simulink model "sgMdl_IO291_HS_DigitalLoopback"  (R2024b)
settings: Solver=FixedStepAuto  StartTime=0.0  StopTime=inf  RelTol=1e-3  EnableMultiTasking=on
undefined symbols (not defined in the file): HS, IO291
libraries: speedgoatlib_IO291 x5
Description:
  | IO291 HighSide - Digital LVTTL and FET Loopback
settings Model: ModifiedByFormat=Speedgoat  SimulationMode=external  ExtModeTrigDuration=100000  Creator=Speedgoat  LastModifiedBy=Speedgoat
settings SolverCC: ConcurrentTasks=on  AlgebraicLoopSolver=TrustRegion  PositivePriorityOrder=on  AutoInsertRateTranBlk=on
settings DataIOCC: LimitDataPoints=on  SaveFormat=StructureWithTime  ReturnWorkspaceOutputs=off
settings OptimizationCC: BlockReduction=off  OptimizeBlockIOStorage=off  BufferReuse=off  ReuseModelBlockBuffer=off  GlobalBufferReuse=off  ExpressionFolding=off  LocalBlockOutputs=off  OptimizeDataStoreBuffers=off  BusAssignmentInplaceUpdate=off
settings DebuggingCC: TasksWithSamePriorityMsg=none  UnconnectedInputMsg=warning  UnconnectedOutputMsg=warning  UnconnectedLineMsg=warning  AllowSymbolicDim=off  SFUnexpectedBacktrackingDiag=warning  SFNoUnconditionalDefaultTransitionDiag=warning  ArithmeticOperatorsInVariantConditions=warning
settings HardwareCC: ProdBitPerLong=64  ProdLongLongMode=on  ProdHWDeviceType=Intel->x86-64 (Linux 64)
settings ModelReferenceCC: EnableRefExpFcnMdlSchedulingChecks=on  PropagateSignalLabelsOutOfModel=off
settings SFSimCC: SimUseLocalCustomCode=off  CustomCodeUndefinedFunction=UseInterfaceOnly
settings RTWCC: Description=Speedgoat Real-Time Target Machine  SystemTargetFile=speedgoat.tlc  TemplateMakefile=slrealtime_default_tmf  RTWUseLocalCustomCode=off  Toolchain=Simulink Real-Time Toolchain  BuildConfiguration=Faster Runs  TargetLang=C++  GPUComputeCapability=3.5  DLArmComputeVersion=19.05
settings CodeAppCC: StateflowObjectComments=on
settings SimulinkRealTimeTargetCC: SubcomponentCodeInterfacePackaging=Reusable function  InstructionSetFMA=off  LogToMDFFile=off  SLRTFileLogMaxRuns=10  UseGCCFastMath=on
settings ConfigComp: CovMetricSettings=dw  CovSaveCumulativeToWorkspaceVar=on  CovSaveSingleToWorkspaceVar=on  CovExternalEMLEnable=off  CovBoundaryAbsTol=1.0e-5

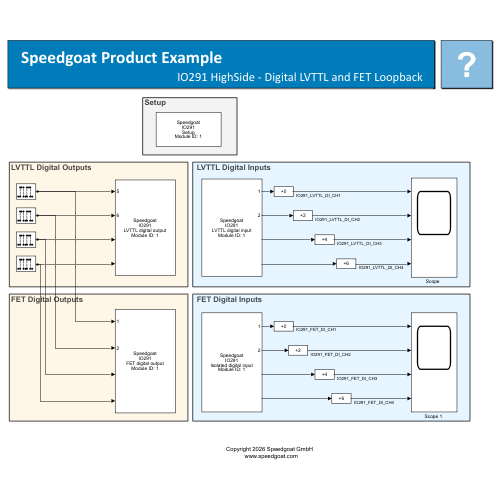
[thumbnail: Simulink's stored preview of the top-level diagram]
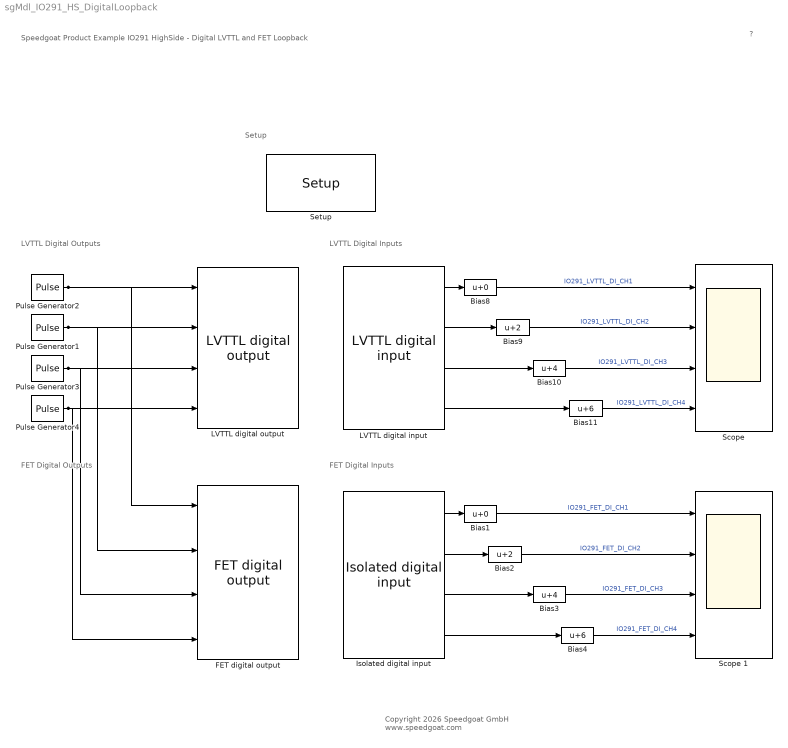
== system sgMdl_IO291_HS_DigitalLoopback ==
  note: LVTTL Digital Outputs
  note: LVTTL Digital Inputs
  note: Setup
  note: FET Digital Outputs
  note: FET Digital Inputs
  note: Speedgoat Product Example
      | IO291 HighSide - Digital LVTTL and FET Loopback
  note: ?
  note: Copyright 2026 Speedgoat GmbH
      |  www.speedgoat.com
  Bias1 : Bias  SaturateOnIntegerOverflow=off
  Bias10 : Bias  Bias=4  SaturateOnIntegerOverflow=off
  Bias11 : Bias  Bias=6  SaturateOnIntegerOverflow=off
  Bias2 : Bias  Bias=2  SaturateOnIntegerOverflow=off
  Bias3 : Bias  Bias=4  SaturateOnIntegerOverflow=off
  Bias4 : Bias  Bias=6  SaturateOnIntegerOverflow=off
  Bias8 : Bias  SaturateOnIntegerOverflow=off
  Bias9 : Bias  Bias=2  SaturateOnIntegerOverflow=off
  "FET digital output " : speedgoatlib_IO291/FET digital output   parModuleId=1  parSampleTime=0.01  parPortConf=1 port for each active output channel  parPciSlot=-1  parFetDoChannels=[1 2 3 4]  parFetDoInitValues=[0 0 0 0]  parFetDoReset=[1 1 1 1]  parModuleType=IO291-HS  parInternalModuleId=1
      settings: SourceProductName=Simulink Real-Time: Speedgoat I/O Blockset
  "Isolated digital input " : speedgoatlib_IO291/Isolated digital input   parModuleId=1  parSampleTime=0.01  parPortConf=1 port for each active input channel  parDataType=Double  parPciSlot=-1  parIsolDiChannels=[1 2 3 4]  parModuleType=IO291-HS  parInternalModuleId=1
      settings: SourceProductName=Simulink Real-Time: Speedgoat I/O Blockset
  "LVTTL digital input " : speedgoatlib_IO291/LVTTL digital input   parModuleId=1  parSampleTime=0.01  parPortConf=1 port for each active input channel  parDataType=Double  parPciSlot=-1  parTtlDiChannels=[1 2 3 4]  parModuleType=IO291-HS  parInternalModuleId=1
      settings: SourceProductName=Simulink Real-Time: Speedgoat I/O Blockset
  "LVTTL digital output " : speedgoatlib_IO291/LVTTL digital output   parModuleId=1  parSampleTime=0.01  parPortConf=1 port for each active output channel  parPciSlot=-1  parTtlDoChannels=[5 6 7 8]  parTtlDoInitValues=[0 0 0 0]  parTtlDoReset=[1 1 1 1]  parModuleType=IO291-HS  parInternalModuleId=1
      settings: SourceProductName=Simulink Real-Time: Speedgoat I/O Blockset
  Pulse Generator1 : DiscretePulseGenerator  Period=10  PulseWidth=4  SampleTime=0.01
  Pulse Generator2 : DiscretePulseGenerator  Period=10  PulseWidth=2  SampleTime=0.01
  Pulse Generator3 : DiscretePulseGenerator  Period=10  PulseWidth=6  SampleTime=0.01
  Pulse Generator4 : DiscretePulseGenerator  Period=10  PulseWidth=8  SampleTime=0.01
  "Scope  " : Scope  NumInputPorts=4
  "Scope 1 " : Scope  NumInputPorts=4
  "Setup " : speedgoatlib_IO291/Setup   parInternalModuleId=1  parPciSlot=-1  parModuleId=1  parModuleType=IO291-HS  parTtlDoChannels=[5:8]  parTtlDoInitValues=0  parTtlDoReset=1  parTtlDiChannels=[1:4]  parIsolDiChannels=[1:4]  parFetDoChannels=[1:4]  parFetDoInitValues=0  parFetDoReset=1
      settings: SourceProductName=Simulink Real-Time: Speedgoat I/O Blockset
  wires:
  "Isolated digital input "/4 -> Bias4/1
  "Isolated digital input "/3 -> Bias3/1
  "Isolated digital input "/2 -> Bias2/1
  "Isolated digital input "/1 -> Bias1/1
  "LVTTL digital input "/4 -> Bias11/1
  "LVTTL digital input "/3 -> Bias10/1
  "LVTTL digital input "/2 -> Bias9/1
  "LVTTL digital input "/1 -> Bias8/1
  Pulse Generator4/1 -> "FET digital output "/4, "LVTTL digital output "/4
  Pulse Generator3/1 -> "LVTTL digital output "/3, "FET digital output "/3
  Pulse Generator1/1 -> "FET digital output "/2, "LVTTL digital output "/2
  Pulse Generator2/1 -> "FET digital output "/1, "LVTTL digital output "/1
  Bias8/1 -> "Scope  "/1  "IO291_LVTTL_DI_CH1"
  Bias9/1 -> "Scope  "/2  "IO291_LVTTL_DI_CH2"
  Bias10/1 -> "Scope  "/3  "IO291_LVTTL_DI_CH3"
  Bias11/1 -> "Scope  "/4  "IO291_LVTTL_DI_CH4"
  Bias1/1 -> "Scope 1 "/1  "IO291_FET_DI_CH1"
  Bias2/1 -> "Scope 1 "/2  "IO291_FET_DI_CH2"
  Bias3/1 -> "Scope 1 "/3  "IO291_FET_DI_CH3"
  Bias4/1 -> "Scope 1 "/4  "IO291_FET_DI_CH4"
